simulink library "etherlab_lib_exp"  (Simulink 6.5)
undefined symbols (not defined in the file or in its folder): catch_check
settings Model: Creator=rich  LastModifiedBy=ml  ExtModeAutoUpdateStatusClock=off

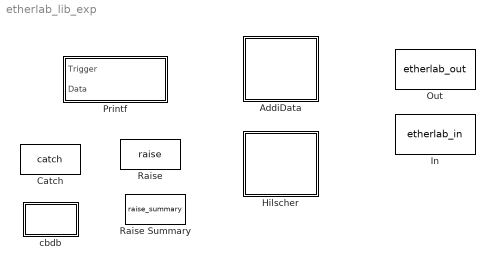
== system etherlab_lib_exp ==
  AddiData : Subsystem
  Catch : S-Function  InitFcn=catch_check(gcb,'CheckIds');  FunctionName=catch  Parameters=ErrId,dtype,Width,TSample  mask{ErrId=E10, dtype=boolean, TSample=0, Width=0, SrcPath=0, SrcCount=0}
      mask prompts: ErrId "Error Identifier"; dtype "Output Data Type Mode"; TSample "Sample Time (-1 inherited)"; SrcPath "Source Paths (Info only)"; SrcCount "Source Count"
      mask StyleString: edit,popup(double|single|int8|uint8|int16|uint16|int32|uint32|boolean|Inherit via back propagation),edit,edit,edit,edit
      mask CallbackString: catch_check(gcb,'CheckIds');|||||
      mask Display: fprintf('%s',ErrId);
  Hilscher : Subsystem
  In : S-Function  FunctionName=etherlab_in  Parameters=varname,src_dtype,len,scale,offset,out_dtype,tsample  mask(Generic Output Port){varname='SIG01', src_dtype=boolean, len=1, scale=0, offset=0, out_dtype=Same as Source, tsample=0}
      mask prompts: varname "Signal Name"; src_dtype "Source Data Type"; len "Array Length"; scale "Output Scale"; offset "Output Offset"; out_dtype "Block Output Data Type"; tsample "Sample Time (-1 for inherited)"
      mask StyleString: edit,popup(boolean|int8|uint8|int16|uint16|int32|uint32|single|double),edit,edit,edit,popup(Same as Source|Double|Double with Scale and Offset),edit
      mask Display: fprintf(varname)
  Out : S-Function  FunctionName=etherlab_out  Parameters=varname,dtype,tsample  mask(Generic Output Port){varname='SIG01', dtype=Inherited, tsample=-1}
      mask prompts: varname "Signal Name"; dtype "Output Data Type"; tsample "Sample Time (-1 for inherited)"
      mask StyleString: edit,popup(Inherited|boolean|int8|uint8|int16|uint16|int32|uint32|int64|uint64|single|double),edit
      mask Display: fprintf(varname)
  Printf : Subsystem  mask{format=0}
      mask prompts: format "Format String"
  Raise : S-Function  FunctionName=raise  Parameters=ErrId,ErrStr,TSample  mask{ErrId=E10, ErrStr=Voltage Too High, TSample=-1, DstPath=0, DstCount=0}
      mask prompts: ErrId "Error Identifier"; ErrStr "Error String"; TSample "Sample Time (-1 inherited)"; DstPath "Destination Paths"; DstCount "Destination Count"
      settings: CopyFcn=raise_check(gcb,'CheckCopy');
      mask CallbackString: raise_check(gcb,'CheckId');||||
      mask Display: fprintf('%s',ErrId);
  Raise Summary : S-Function  FunctionName=raise_summary  Parameters=ErrId,ErrStr,ErrSrc,DstPath  mask{ErrId=E1x, ErrStr=Voltage Too High, ErrSrc=E10, DstPath=0}
      mask prompts: ErrId "Error Identifier"; ErrStr "Error String"; ErrSrc "Error Sources"; DstPath "Destination Paths"
      settings: CopyFcn=raise_summary_check(gcb,'CheckCopy');
      mask Display: fprintf('%s\n%s',ErrId,ErrSrc);
  cbdb : Subsystem  LoadFcn=|  InitFcn=|  StartFcn=|  StopFcn=|  ClipboardFcn=|
      | if ~strcmp(gcs,'rtai_lib')
      | display('LoadFcn');       
      | end
      | if ~strcmp(gcs,'rtai_lib')
      | display('InitFcn');       
      | end
      | if ~strcmp(gcs,'rtai_lib')
      | display('StartFcn');      
      | end
      | if ~strcmp(gcs,'rtai_lib')
      | display('StopFcn');       
      | end
      | if ~strcmp(gcs,'rtai_lib')
      | display('ClipboardFcn');  
      | end
      settings: CopyFcn=|
      | if ~strcmp(gcs,'rtai_lib')
      | display('CopyFcn');
      | end
      settings: DeleteFcn=|
      | if ~strcmp(gcs,'rtai_lib')
      | display('DeleteFcn');
      | end
      settings: UndoDeleteFcn=|
      | if ~strcmp(gcs,'rtai_lib')
      | display('UndoDeleteFcn');
      | end
      settings: ModelCloseFcn=|
      | if ~strcmp(gcs,'rtai_lib')
      | display('ModelCloseFcn');
      | end
      settings: PreSaveFcn=|
      | if ~strcmp(gcs,'rtai_lib')
      | display('PreSaveFcn');
      | end
      settings: PostSaveFcn=|
      | if ~strcmp(gcs,'rtai_lib')
      | display('PostSaveFcn');
      | end
      settings: NameChangeFcn=|
      | if ~strcmp(gcs,'rtai_lib')
      | display('NameChangeFcn');
      | end
      settings: DestroyFcn=|
      | if ~strcmp(gcs,'rtai_lib')
      | display('DestroyFcn');
      | end
      settings: OpenFcn=|
      | if ~strcmp(gcs,'rtai_lib')
      | display('OpenFcn');
      | end
      settings: CloseFcn=|
      | if ~strcmp(gcs,'rtai_lib')
      | display('CloseFcn');
      | end
      settings: ParentCloseFcn=|
      | if ~strcmp(gcs,'rtai_lib')
      | display('ParentCloseFcn');
      | end
      settings: MoveFcn=|
      | if ~strcmp(gcs,'rtai_lib')
      | display('MoveFcn');
      | end
      mask Display: disp('Callback\nDebugger');

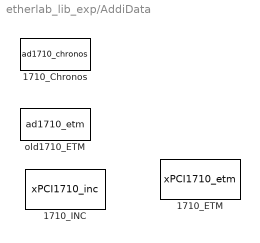
== system etherlab_lib_exp/AddiData ==
  1710_Chronos : S-Function  FunctionName=ad1710_chronos  Parameters=b_BoardHandle,b_ModuleNumber,b_ChronoMode,b_PCIInputClock,b_TimeUnit,ul_TimeOut,b_TimeoutUnit  mask{b_BoardHandle=0, b_ModuleNumber=0, b_ChronoMode=0, b_PCIInputClock=30MHz, b_TimeUnit=Microseconds, ul_TimeOut=0, b_TimeoutUnit=Micoseconds}
      mask prompts: b_BoardHandle "Board Handle"; b_ModuleNumber "Module Number"; b_ChronoMode "Chrono Mode"; b_PCIInputClock "PCI Input Clock"; b_TimeUnit "Time Unit"; ul_TimeOut "Timeout"; b_TimeoutUnit "Timeout Unit"
      mask StyleString: edit,popup(0|1|2|3),popup(0|1|2|3|4|5|6|7),popup(30MHz|33MHz|40MHz),popup(Nanoseconds|Microseconds|Milliseconds|Seconds|Minutes),edit,popup(Nanoseconds|Micoseconds|Milliseconds|Seconds|Minutes)
      mask Display:
      | fprintf('1710 Chrono\nB:%i M/d:%i',
      | b_BoardHandle,b_ModuleNumber);
  1710_ETM : S-Function  FunctionName=xPCI1710_etm  Parameters=device,module,clock_src,divisor,op_type,tsample  mask(Addi Data 1710 ETM){device=01:0A, module=0, clock_src=Internal 40MHz, divisor=1, op_type=double, scale=0, offset=0, tsample=0}
      mask prompts: device "PCI Device"; module "Module Number"; clock_src "Clock Source"; divisor "Clock Divisor"; op_type "Output Data Type"; scale "Output Full Scale"; offset "Output Offset"; tsample "Sampling Time (-1 inherited)"
      mask help: This block implements the Edge Triggered Timer Mode for the 1710 Addi Data timer card.
      mask init:
      | device = test_var(device);
      mask StyleString: edit,popup(0|1|2|3),popup(Internal 40MHz|PCI Bus 33/30Mhz),edit,popup(double|single|int8|uint8|int16|uint16|int32|uint32|boolean|Inherited via back propagation),edit,edit,edit
      mask Display:
      | fprintf('xPCI1710 ETM\nPCI: %s\nModule: %i',
      | device,module-1);
  1710_INC : S-Function  FunctionName=xPCI1710_inc  Parameters=device,module,mode,width,op_type,preset,tsample  mask(Addi Data 1710 INC){device=03:0E, module=0, mode=Quadruple, width=32-Bit, op_type=double, preset=off, tsample=0}
      mask prompts: device "PCI Device"; module "Module Number"; width "Counter Width"; op_type "Output Data Type"; preset "Preset Input"; tsample "Sampling Time (-1 inherited)"
      mask help: This block implements the Incremental Counter Mode for the 1710 Addi Data timer card.
      mask init:
      | device = test_var(device);
      mask StyleString: edit,popup(0|1|2|3),popup(Quadruple|Double|Simple|Direct),popup(32-Bit|16-Bit),popup(double|single|int8|uint8|int16|uint16|int32|uint32|boolean|Inherited via back propagation),checkbox,edit
      mask Display:
      | fprintf('xPCI1710 INC\nPCI: %s\nModule: %i',
      | device,module-1);
  old1710_ETM : S-Function  FunctionName=ad1710_etm  Parameters=b_BoardHandle,b_ModuleNumber,b_ClockSelection,b_TimingUnit,ul_Timing  mask(Addi Data 1710 ETM){b_BoardHandle=0, b_ModuleNumber=0, b_ClockSelection=PCI 30MHz, b_TimingUnit=Microseconds, ul_Timing=0}
      mask prompts: b_BoardHandle "Board Handle"; b_ModuleNumber "Module Number"; b_ClockSelection "Clock Selection"; b_TimingUnit "Timing Unit"; ul_Timing "Time Base"
      mask help:
      | This block implements the Edge Triggered Mode for the 1710 Addi Data timer card.
      |
      | Both counters are exported as a vector.
      mask StyleString: edit,popup(0|1|2|3),popup(PCI 30MHz|PCI 33MHz|Internal 40MHz),popup(Nanoseconds|Microseconds|Milliseconds),edit
      mask Display:
      | fprintf('1710 ETM\nB:%i M/d:%i',
      | b_BoardHandle,b_ModuleNumber);

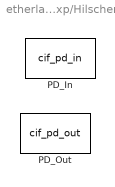
== system etherlab_lib_exp/Hilscher ==
  PD_In : S-Function  FunctionName=cif_pd_in  Parameters=device,addr,ip_type,width,swap,op_type,tsample  mask(Profibus Input){device=01:0E, addr=120, ip_type=int8_T, width=8, swap=off, op_type=int8, tsample=0}
      mask prompts: device "PCI Device"; addr "Address"; ip_type "Sensor Data Type"; width "Vector Length"; swap "Swap Input Bytes"; op_type "Output Data Format"; tsample "Sample Time (-1 inherited)"
      mask help: Hilscher CIF-80PB Profibus Input
      mask init:
      | device = test_var(device);
      mask Help:
      | This block provides an interface to the Profibus incoming process image for the Hilscher CIF-80PB Card.
      | <p>
      | Supply the following information:<br>
      | <b>PCI Device</b>: Either supply the address in PCI-Addressing format <em>bus:slot</em> (hexadecimal format), or the (decimal) position as cards are detected
      mask StyleString: edit,edit,popup(Bit0|Bit1|Bit2|Bit3|Bit4|Bit5|Bit6 |Bit7|int8_T|uint8_T|int16_T|uint16_T|int32_T|uint32_T),edit,checkbox,popup(int8|uint8|int16|uint16|int32|uint32|boolean|double|single|Inherited via back propagation),edit
      mask Display:
      | fprintf('CIF-80PB\nPCI: %s\nAddr:%i',
      | device,addr);
  PD_Out : S-Function  FunctionName=cif_pd_out  Parameters=device,addr,op_type,swap,tsample  mask(Profibus Input){device=01:0E, addr=120, op_type=int8_T, swap=off, tsample=-1}
      mask prompts: device "PCI Device"; addr "Address"; op_type "Actuator Data Type"; swap "Swap Input Bytes"; tsample "Sample Time (-1 inherited)"
      mask help: Hilscher CIF-80PB Profibus Output
      mask init:
      | device = test_var(device);
      mask Help:
      | This block provides an interface to the Profibus outgoing process image for the Hilscher CIF-80PB Card.
      | <p>
      | Supply the following information:<br>
      | <b>PCI Device</b>: Either supply the address in PCI-Addressing format <em>bus:slot</em> (hexadecimal format), or the (decimal) position as cards are detected
      mask StyleString: edit,edit,popup(Bit0|Bit1|Bit2|Bit3|Bit4|Bit5|Bit6 |Bit7|int8_T|uint8_T|int16_T|uint16_T|int32_T|uint32_T),checkbox,edit
      mask Display:
      | fprintf('CIF-80PB\nPCI: %s\nAddr:%i',
      | device,addr);

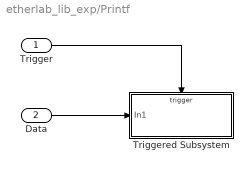
== system etherlab_lib_exp/Printf ==
  Trigger : Inport
  Data : Inport  Port=2
  Triggered Subsystem : Subsystem  TreatAsAtomicUnit=on
  wires:
  Trigger/1 -> Triggered Subsystem/Trigger
  Data/1 -> Triggered Subsystem/1(In1)

== system etherlab_lib_exp/cbdb ==

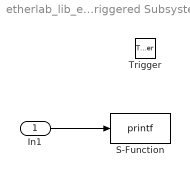
== system etherlab_lib_exp/Printf/Triggered Subsystem ==
  In1 : Inport
  Trigger : TriggerPort
  S-Function : S-Function  FunctionName=printf  Parameters=format
  wires:
  In1/1 -> S-Function/1
